simulink model "robot_prototype_simulation"  (R2022b)
settings: Solver=VariableStepAuto  StartTime=0.0  StopTime=10.0  RelTol=1e-3
values from neighbouring files (symbols this model uses):
  T_S = 10e-3    (= 0.01)    [robot_prototype_init.m]
settings Model: Creator=hp  LastModifiedBy=hp

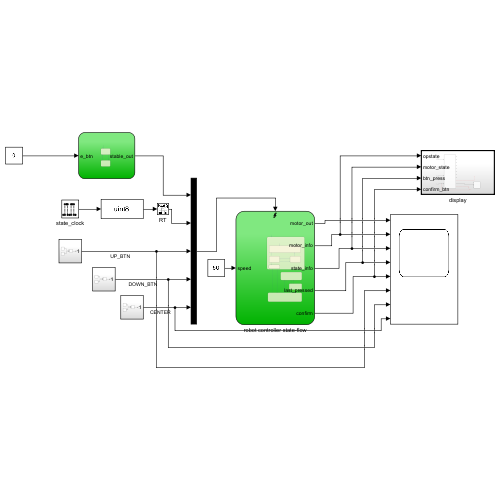
[thumbnail: Simulink's stored preview of the top-level diagram]
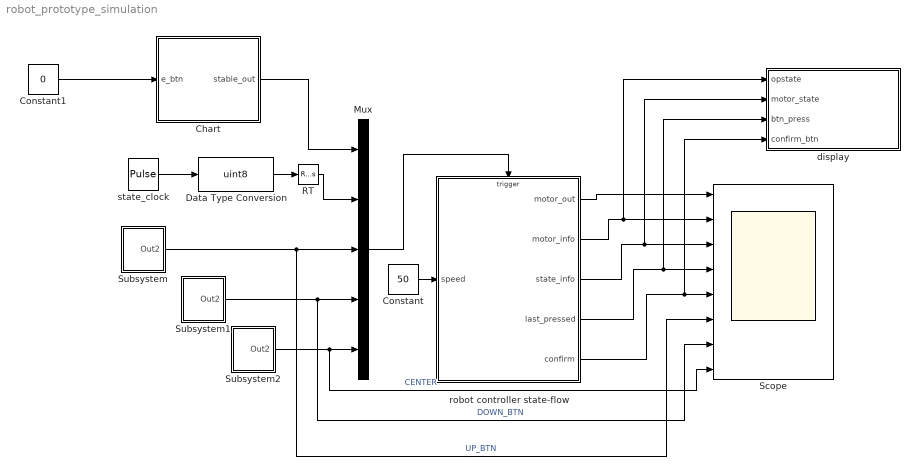
== system robot_prototype_simulation ==
  Chart : Stateflow chart  TreatAsAtomicUnit=on
  Constant : Constant  Value=50
  Constant1 : Constant  Value=0  OutDataTypeStr=uint8
  Data Type Conversion : DataTypeConversion  OutMin=0  OutMax=255  OutDataTypeStr=uint8  SaturateOnIntegerOverflow=off  RndMeth=Floor
  Mux : Mux  Inputs=5
  RT : RateTransition  OutPortSampleTime=T_S
  Scope : Scope  NumInputPorts=8
  Subsystem : Subsystem
  Subsystem1 : Subsystem
  Subsystem2 : Subsystem
  display : Subsystem  TreatAsAtomicUnit=on
  robot controller state-flow : Stateflow chart  TreatAsAtomicUnit=on
  state_clock : DiscretePulseGenerator  Period=100  PulseWidth=50  PhaseDelay=20  SampleTime=T_S
  wires:
  robot controller state-flow/3(state_info) -> display/2(motor_state), Scope/3
  RT/1 -> Mux/2
  robot controller state-flow/5(confirm) -> display/4(confirm_btn), Scope/5
  Subsystem2/1(Out2) -> Scope/8, Mux/5  "CENTER"
  Chart/1(stable_out) -> Mux/1
  Mux/1 -> robot controller state-flow/Trigger
  robot controller state-flow/1(motor_out) -> Scope/1
  Subsystem/1(Out2) -> Scope/6, Mux/3  "UP_BTN"
  robot controller state-flow/4(last_pressed) -> display/3(btn_press), Scope/4
  Constant/1 -> robot controller state-flow/1(speed)
  Data Type Conversion/1 -> RT/1
  Constant1/1 -> Chart/1(e_btn)
  state_clock/1 -> Data Type Conversion/1
  robot controller state-flow/2(motor_info) -> display/1(opstate), Scope/2
  Subsystem1/1(Out2) -> Scope/7, Mux/4  "DOWN_BTN"

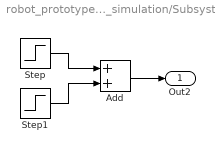
== system robot_prototype_simulation/Subsystem ==
  Add : Sum  OutDataTypeStr=uint8
  Step : Step  SampleTime=0
  Step1 : Step  Time=1.5  After=-1  SampleTime=0
  Out2 : Outport
  wires:
  Step/1 -> Add/1
  Step1/1 -> Add/2
  Add/1 -> Out2/1

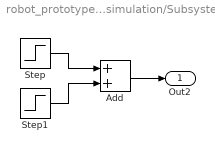
== system robot_prototype_simulation/Subsystem1 ==
  Add : Sum  OutDataTypeStr=uint8
  Step : Step  Time=5  SampleTime=0
  Step1 : Step  Time=5.5  After=-1  SampleTime=0
  Out2 : Outport
  wires:
  Add/1 -> Out2/1
  Step1/1 -> Add/2
  Step/1 -> Add/1

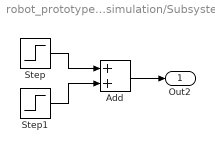
== system robot_prototype_simulation/Subsystem2 ==
  Add : Sum  OutDataTypeStr=uint8
  Step : Step  Time=3  SampleTime=0
  Step1 : Step  Time=3.5  After=-1  SampleTime=0
  Out2 : Outport
  wires:
  Step/1 -> Add/1
  Step1/1 -> Add/2
  Add/1 -> Out2/1

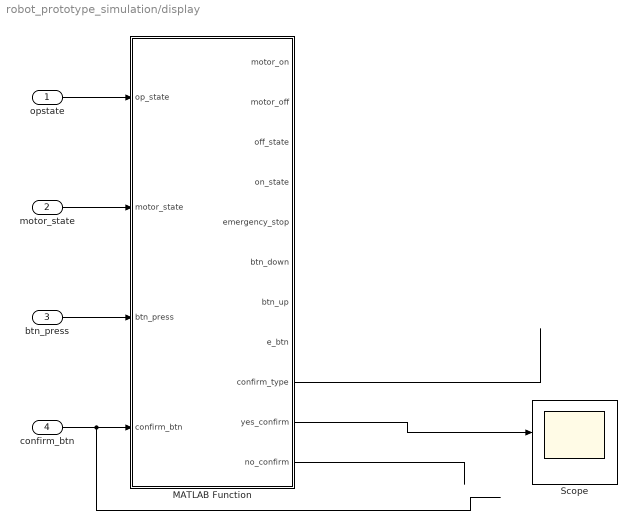
== system robot_prototype_simulation/display ==
  opstate : Inport
  motor_state : Inport  Port=2
  btn_press : Inport  Port=3
  confirm_btn : Inport  Port=4
  MATLAB Function : MATLAB Function  TreatAsAtomicUnit=on
  Scope : Scope  NumInputPorts=4
  wires:
  opstate/1 -> MATLAB Function/1(op_state)
  motor_state/1 -> MATLAB Function/2(motor_state)
  btn_press/1 -> MATLAB Function/3(btn_press)
  confirm_btn/1 -> MATLAB Function/4(confirm_btn)
  MATLAB Function/10(yes_confirm) -> Scope/2
  MATLAB Function/11(no_confirm) -> ?
  MATLAB Function/9(confirm_type) -> ?

== stateflow chart robot_prototype_simulation/Chart ==
  state off
    entry:
    stable_out = 0
  note: ]
  state on
    entry:
    stable_out = 1
  (default) -> off
  on -> off : [duration(e_btn<0.3) > 20e-3]
  off -> on : [duration(e_btn> 0.7) > 20e-3]
  data: e_btn input; stable_out output uint8

== matlab function robot_prototype_simulation/display/MATLAB Function ==
  data: op_state input; motor_on output; motor_off output; motor_state input; off_state output; on_state output; emergency_stop output; btn_down output; btn_up output; e_btn output; btn_press input; confirm_btn input; confirm_type output; yes_confirm output; no_confirm output
function [motor_on,motor_off, off_state, on_state, emergency_stop, btn_down, btn_up ,e_btn , confirm_type ,yes_confirm, no_confirm] = fcn(op_state, motor_state, btn_press, confirm_btn)

motor_on = 0;
motor_off = 0;

off_state = 0;
on_state = 0;
emergency_stop = 0;

btn_down = 0;
btn_up = 0;
e_btn = 0;

confirm_type = 0;
yes_confirm = 0;
no_confirm = 0;
% for displaying motor state
if motor_state == 0
    motor_off = 1;
elseif motor_state == 1
    motor_on = 1;
end

% for displaying states
if op_state == 0
    off_state = 1;
elseif op_state == 1
    on_state = 1;
elseif op_state == 2
    emergency_stop = 1;
end

%for displaying button press
if btn_press == 1
    btn_down = 1;
elseif btn_press == 2
    btn_up = 1;
elseif btn_press == 3
    e_btn = 1;
end

%for displaying which action to confirm
%i.e. either star action or stop action
if confirm_btn == 1 || confirm_btn == 2
    confirm_type = 1;
end
  
if confirm_btn == 1 && confirm_type == 1
    yes_confirm = 1;
elseif confirm_btn == 2 && confirm_type == 1
    no_confirm = 1;
end

== stateflow chart robot_prototype_simulation/robot controller state-flow ==
  state Off_super_state
    entry:
    motor_out = 0;
    motor_info = 0;
    state_info = 0;
    start_robot = 0;
    state state_off
      entry:
      motor_out = 0;
      motor_info = 0;
      state_info = 0;
      confirm = 0;
    state confirm_start_action_
      entry:
      confirm = 1;
    state cancel_start_action
      entry:
      confirm = 2;
    state confirmed_start
      entry:
      start_robot = 1
    (default) -> state_off
    state_off -> confirm_start_action_ : up_btn{button_type = 2}
    cancel_start_action -> state_off [order 1] : center_btn{confirm = 0}
    cancel_start_action -> confirm_start_action_ [order 2] : up_btn
    confirm_start_action_ -> cancel_start_action [order 2] : down_btn
    confirm_start_action_ -> confirmed_start [order 1] : center_btn
  note: button_type is internal variable used to store which button was pressed
      | 0 = no button press
      | 1 = down
      | 2 = up
      | 3 = emergency_button
      | 4 = center_button
  note: These confirmation applies when confirming to turn on the robot
      |
      | confirm = 1
      | display 1 at the confirm position
      | confirm = 2
      | display 1 at cancel position
      |
      | 0
      | anything else don't display anything.
  state emergency_stop
    entry:
    motor_out = 0;
    motor_info = 0;
    state_info = 2;
    last_pressed = button_type;
  state intermediate
  note: emergency_btn
  state go
    entry:
    confirm = 0;
    motor_out = speed;
    motor_info = 1;
    state_info = 1;
    last_pressed = button_type;
  (default) -> Off_super_state
  go -> Off_super_state [order 2] : down_btn{button_type = 1;
      | start_robot = 0;}
  Off_super_state -> go : [start_robot == 1]{button_type = 4;confirm = 0;}
  go -> emergency_stop [order 1] : emergency_btn{button_type = 3}
  emergency_stop -> intermediate : emergency_btn
  intermediate -> emergency_stop [order 1] : after(0.5, sec)
  intermediate -> go [order 2]
  data: motor_out output; speed input; motor_info output; state_info output; button_type local =0; last_pressed output; confirm output; start_robot local =0
  events: emergency_btn input RISING_EDGE_EVENT; active_chart input RISING_EDGE_EVENT; up_btn input RISING_EDGE_EVENT; down_btn input RISING_EDGE_EVENT; center_btn input RISING_EDGE_EVENT
